simulink model "untitled1"  (R2021a)
settings: Solver=VariableStepAuto  StartTime=0.0  StopTime=10.0  RelTol=1e-3
settings Model: Creator=yusuke  LastModifiedBy=yusuke

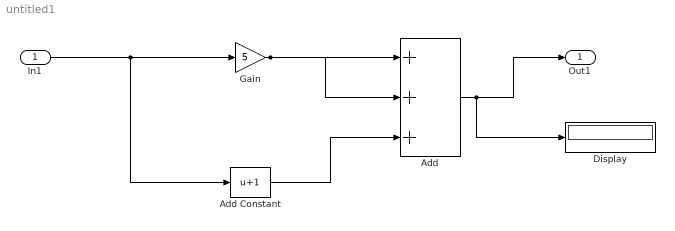
== system untitled1 ==
  In1 : Inport
  Add : Sum  Inputs=+++
  Add Constant : Bias  Bias=1
  Display : Display
  Gain : Gain  Gain=5
  Out1 : Outport
  wires:
  In1/1 -> Add Constant/1, Gain/1
  Add/1 -> Display/1, Out1/1
  Gain/1 -> Add/1, Add/2
  Add Constant/1 -> Add/3
